simulink model "matrixMultEigenTest"  (R2013b)
settings: Solver=ode3  StartTime=0.0  StopTime=1  FixedStep=0.001  RelTol=1e-3
InitFcn:
  | dim = 80;
  | dimMatrix = randn(dim,dim);
  | 
  | disp( sprintf('\ndimension to test is dim = %i',dim) )
StopFcn:
  | disp('');
  | len = size(original.Data);
  | valid = 1;
  | 
  | biggestError = 0;
  | 
  | for k=1:len
  |   temp = abs(original.Data(:,:,k) - own.Data(:,:,k)) > 1e-10;
  |   temp1 = max( max(abs(original.Data(:,:,k) - own.Data(:,:,k))) );
  | 
  |   if( temp1 > biggestError )
  |     biggestError = temp1;
  |   end
  | 
  |   if( any(any( temp ) ) )
  |     error('mismatch during comparison')
  |     valid = 0;
  |     break;
  |   end
  | end
  | 
  | if( valid == 1 )
  |   disp('no mismatch found!')
  |   disp( sprintf('greatest deviation is %f*1e-13', biggestError*1e13) )
  | end
settings Model: Creator=rtai-ao  LastModifiedBy=rtai-ao
settings RTWCC: SystemTargetFile=rtai.tlc  TemplateMakefile=rtai.tmf  Description=Linux RTAI Real-Time Target  GenerateReport=on  ProcessScript=rtai_make_rtw_hook  BuildConfiguration=Faster Runs
settings STFCustomTargetCC: ModelReferenceCompliant=off  GeneratePreprocessorConditionals=Disable all  MatFileLogging=on  MATLABClassNameForMDSCustomization=Simulink.SoftwareTarget.TargetSpecificTriggerConfigurationBase  SystemTargetFile=rtai.tlc

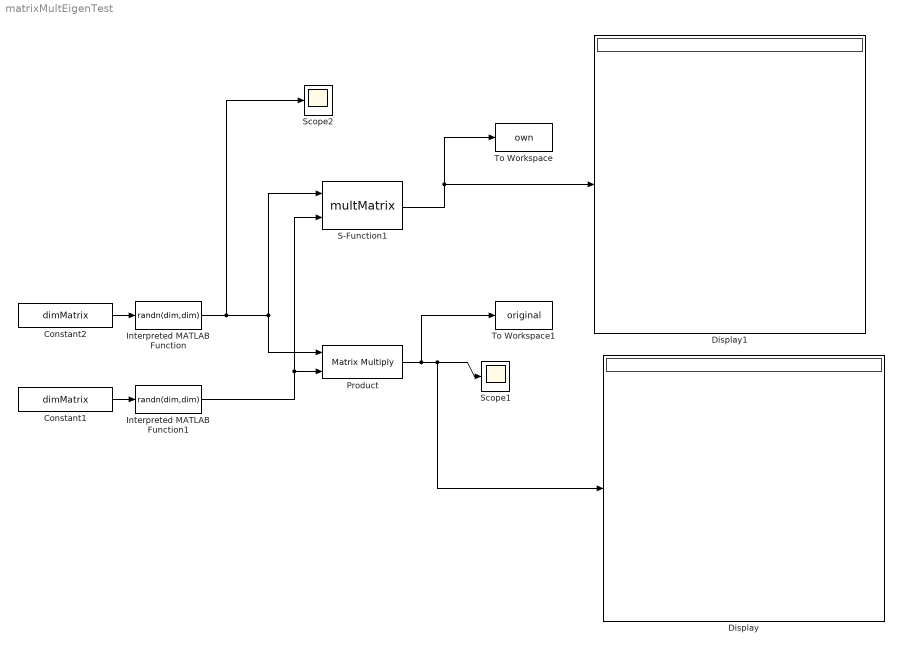
== system matrixMultEigenTest ==
  Constant1 : Constant  Value=dimMatrix  VectorParams1D=off
  Constant2 : Constant  Value=dimMatrix  VectorParams1D=off
  Display : Display
  Display1 : Display
  Interpreted MATLAB Function : MATLABFcn  MATLABFcn=randn(dim,dim)  Output1D=off
  Interpreted MATLAB Function1 : MATLABFcn  MATLABFcn=randn(dim,dim)  Output1D=off
  Product : Product  Multiplication=Matrix(*)
  S-Function1 : S-Function  RequirementInfo={} %GIDa_0602442c_123d_45d0_8dfb_a898fe105d51  FunctionName=multMatrix  EnableBusSupport=off
      mask Display:
      | port_label('input',1,'A')
      | port_label('input',2,'B')
      | port_label('output',1,'Y')
      | fprintf('Y=A*B\nEigen3')
  Scope1 : Scope
  Scope2 : Scope
  To Workspace : ToWorkspace  VariableName=own  SampleTime=-1  SaveFormat=Timeseries
  To Workspace1 : ToWorkspace  VariableName=original  SampleTime=-1  SaveFormat=Timeseries
  wires:
  Interpreted MATLAB Function/1 -> Scope2/1, S-Function1/1, Product/1
  Product/1 -> To Workspace1/1, Display/1, Scope1/1
  Interpreted MATLAB Function1/1 -> S-Function1/2, Product/2
  S-Function1/1 -> To Workspace/1, Display1/1
  Constant2/1 -> Interpreted MATLAB Function/1
  Constant1/1 -> Interpreted MATLAB Function1/1
